simulink model "longitudinal_dynamics"  (R2024b)
settings: Solver=VariableStepAuto  StartTime=0.0  StopTime=60  RelTol=1e-2
values from neighbouring files (symbols this model uses):
  Cd = [0 1]    [mpc3.m]
  Cr = 87342    [mpc3.m]    (also in prueba_mpc.m; prueba_mpc2.m)
  Iz = 1960    [mpc3.m]    (also in prueba_mpc.m; prueba_mpc2.m)
  lf = 1.177    [mpc3.m]    (also in prueba_mpc.m; prueba_mpc2.m)
  lr = 1.358    [mpc3.m]    (also in prueba_mpc.m; prueba_mpc2.m)
  m = 1400    [mpc3.m]    (also in prueba_mpc.m; prueba_mpc2.m)
  R = 1    [prueba_mpc.m]    (also in prueba_mpc2.m)
  vx = 10    [mpc3.m]    (also in prueba_mpc.m; prueba_mpc2.m)
undefined symbols (not defined in the file or in its folder): Af, C_lambda, F_max, FN, g, miu, mode, mu1, mu2, mu3, steering_angle, theta
libraries: mpclib x1, slpidlib x1
settings Model: Creator=inaki  LastModifiedBy=inaki

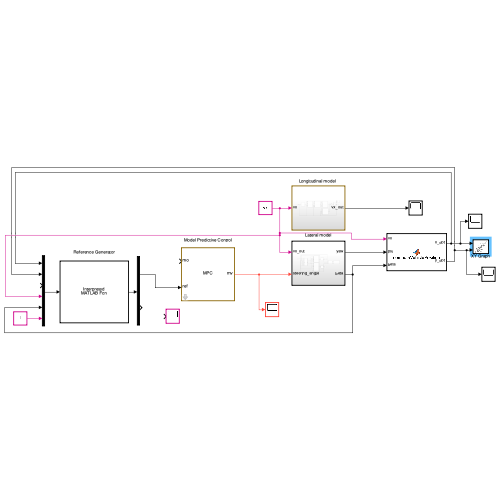
[thumbnail: Simulink's stored preview of the top-level diagram]
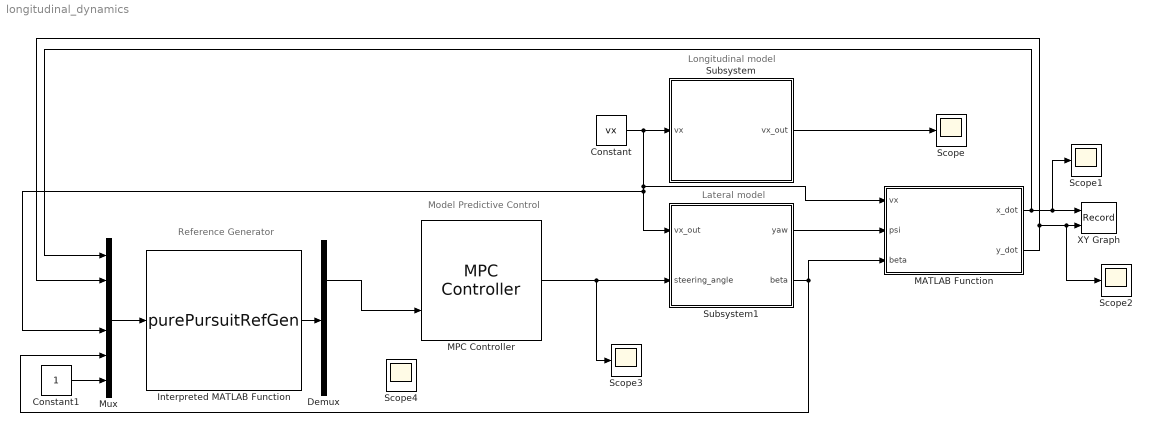
== system longitudinal_dynamics ==
  note: Longitudinal model
  note: Lateral model
  note: Model Predictive Control
  note: Reference Generator
  Constant : Constant  Value=vx
  Constant1 : Constant
  Demux : Demux  Outputs=2
  Interpreted MATLAB Function : MATLABFcn  MATLABFcn=purePursuitRefGen
  MATLAB Function : MATLAB Function  TreatAsAtomicUnit=on
  MPC Controller : mpclib/MPC Controller  SCDEnableBlockLinearizationSpecification=on  mpcobj=mpc1  is_multiple=0  enable_value=0  return_u0=off  updateMPCinCallerWorkspace=on  md_inport=off  mv_inport=off  uref_inport=off  return_cost=off  return_mvseq=off  return_qpstatus=off  return_xseq=off  return_state=off  return_ovseq=off  state_inport=off  umin_inport=off  umax_inport=off  ymin_inport=off  ymax_inport=off  cc_inport=off  ywt_inport=off  uwt_inport=off  duwt_inport=off  rhoeps_inport=off  pm_inport=off  MaximumP=10  HorizonChoice=FixedHorizon  n_ts=0.1  n_p=10  n_mv=1  n_md=0  n_ud=0  n_mo=1  n_uo=0  BlockDataType=double  SampleTimeInherited=off  switch_inport=off
  Mux : Mux  Inputs=6
  Scope{,1..4} (5 alike) : Scope
  Subsystem : Subsystem
  Subsystem1 : Subsystem
  XY Graph : Record  FileSettingsInternal="{\"entries\":[{\"content\":{\"excelSettings\":{\"content\":{},\"type\":\"Streamout.ExcelSettings\"}},\"type\":\"Streamout.FileSettingStorage\",\"uuid\":\"\"}],\"packageUris\":[\"http:\\/\\/schema.mathworks.com\\/mf0\\/streamout_blocks\\/R2020a\"],\"version\":\"1.0\"}"  Layout=[1 1]  SignalsInternal="{\"entries\":[{\"content\":{\"signals\":[{\"content\":{\"blockPath\":[],\"dimensions\":[1],\"domain\":\"\",\"lineColor\":\"#a2142f\",\"plots\":[ 1 ],\"port\":1,\"signalID\":1,\"signalName\":\"MATLAB Function:1\"},\"type\":\"RecordBlkView.Signal\",\"uuid\":\"\"},{\"content\":{\"blockPath\":[],\"dimensions\":[1],\"domain\":\"\",\"lineColor\":\"#139fff\",\"plots\":[ 1 ],\"port\":2,\"signalID\":2,\"signalName\":\"MATLAB Function:2\"},\"type\":\"RecordBlkView.Signal\",\"uuid\":\"\"}]},\"type\":\"RecordBlkView.InputSignals\",\"uuid\":\"\"}],\"packageUris\":[\"http:\\/\\/schema.mathworks.com\\/mf0\\/streamout_blocks\\/R2020a\"],\"version\":\"1.0\"}"  VisualizationBindings="{\"xyplotplugin\":{\"info\":[{\"series\":[{\"bindingParametersList\":[{\"parameter\":\"X-Axis\",\"signalID\":1,\"signalName\":\"MATLAB Function:1\"},{\"parameter\":\"Y-Axis\",\"signalID\":2,\"signalName\":\"MATLAB Function:2\"}],\"seriesID\":0}],\"subplotID\":1}]}}"  CompatibilityTag=XY
  wires:
  Constant/1 -> Subsystem1/1(vx_out), Mux/4, MATLAB Function/1(vx), Subsystem/1(vx)
  Subsystem1/1(yaw) -> MATLAB Function/2(psi)
  Subsystem1/2(beta) -> Mux/5, MATLAB Function/3(beta)
  MATLAB Function/2(y_dot) -> Scope2/1, XY Graph/2, Mux/2
  MATLAB Function/1(x_dot) -> Scope1/1, XY Graph/1, Mux/1
  Interpreted MATLAB Function/1 -> Demux/1
  Demux/1 -> MPC Controller/2
  Mux/1 -> Interpreted MATLAB Function/1
  Constant1/1 -> Mux/6
  MPC Controller/1 -> Scope3/1, Subsystem1/2(steering_angle)
  Subsystem/1(vx_out) -> Scope/1

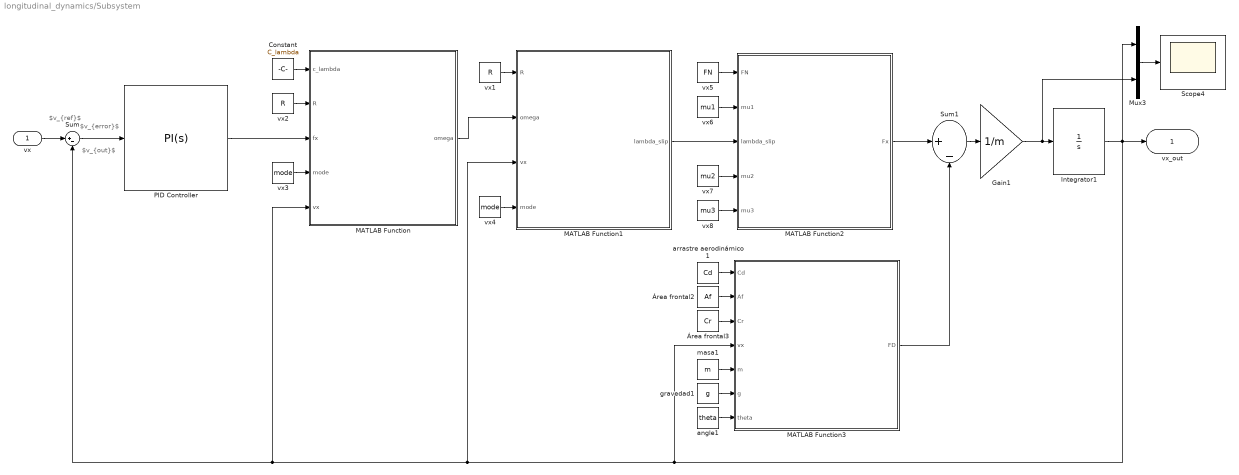
== system longitudinal_dynamics/Subsystem ==
  note: $v_{out}$
  note: $v_{error}$
  note: $v_{ref}$
  vx : Inport
  Constant : Constant  Value=C_lambda
  Gain1 : Gain  Gain=1/m
  Integrator1 : Integrator  ZeroCross=off
  MATLAB Function : MATLAB Function  TreatAsAtomicUnit=on
  MATLAB Function1 : MATLAB Function  TreatAsAtomicUnit=on
  MATLAB Function2 : MATLAB Function  TreatAsAtomicUnit=on
  MATLAB Function3 : MATLAB Function  TreatAsAtomicUnit=on
  Mux3 : Mux  Inputs=2
  PID Controller : slpidlib/PID Controller  Controller=PI  Form=Parallel  TimeDomain=Continuous-time  UseExternalTs=off  SampleTime=-1  IntegratorMethod=Forward Euler  FilterMethod=Forward Euler  ControllerParametersSource=internal  P=3371.8  I=1668.70  UseKiTs=off  D=0  UseExternalDerivativeSource=off  N=100  UseFilter=on  TunerSelectOption=Transfer Function Based (PID Tuner App)  InitialConditionSource=internal  InitialConditionForIntegrator=0  InitialConditionForFilter=0  DifferentiatorICPrevScaledInput=0  ExternalReset=none  TrackingMode=off  Kt=1  LimitOutput=on  SatLimitsSource=internal  UpperSaturationLimit=F_max  LowerSaturationLimit=-F_max  LinearizeAsGain=off  AntiWindupMode=clamping  Kb=1  LimitIntegrator=off  UpperIntegratorSaturationLimit=inf  LowerIntegratorSaturationLimit=-inf  POutMin=[]  POutMax=[]  IOutMin=[]  IOutMax=[]  DOutMin=[]  DOutMax=[]  NOutMin=[]  NOutMax=[]  SumOutMin=[]  SumOutMax=[]  SaturationOutMin=[]  SaturationOutMax=[]  PParamMin=[]  PParamMax=[]  IParamMin=[]  IParamMax=[]  DParamMin=[]  DParamMax=[]  NParamMin=[]  NParamMax=[]  KbParamMin=[]  KbParamMax=[]  KtParamMin=[]  KtParamMax=[]  KbOutMin=[]  KbOutMax=[]  KtOutMin=[]  KtOutMax=[]  IntegratorOutMin=[]  IntegratorOutMax=[]  FilterOutMin=[]  FilterOutMax=[]  SumI1OutMin=[]  SumI1OutMax=[]  SumI2OutMin=[]  SumI2OutMax=[]  SumI3OutMin=[]  SumI3OutMax=[]  SumI4OutMin=[]  SumI4OutMax=[]  SumDOutMin=[]  SumDOutMax=[]  DifferentiatorOutMin=[]  DifferentiatorOutMax=[]  FilterDiffOutCoefMin=[]  FilterDiffOutCoefMax=[]  ReciprocalOutMin=[]  ReciprocalOutMax=[]  SumDenOutMin=[]  SumDenOutMax=[]  SumNumOutMin=[]  SumNumOutMax=[]  DivideOutMin=[]  DivideOutMax=[]  UdiffTsProdOutMin=[]  UdiffTsProdOutMax=[]  NTsProdOutMin=[]  NTsProdOutMax=[]  UintegralTsProdOutMin=[]  UintegralTsProdOutMax=[]  UngainTsProdOutMin=[]  UngainTsProdOutMax=[]  ClampingZeroOutDataTypeStr=Inherit: Inherit via back propagation  ClampingZeroOutMin=[]  ClampingZeroOutMax=[]  FilterDenConstantOutDataTypeStr=Inherit: Inherit via back propagation  FilterDenConstantOutMin=[]  FilterDenConstantOutMax=[]  PCopyOutDataTypeStr=Inherit: Inherit via back propagation  PCopyOutMin=[]  PCopyOutMax=[]  NCopyOutDataTypeStr=Inherit: Inherit via back propagation  NCopyOutMin=[]  NCopyOutMax=[]  IntegratorContinuousStateAttributes=''  IntegratorStateMustResolveToSignalObject=off  IntegratorRTWStateStorageClass=Auto  FilterContinuousStateAttributes=''  FilterStateMustResolveToSignalObject=off  FilterRTWStateStorageClass=Auto  ParallelPVariant=InternalParameters  IdealPVariant=Disabled  IVariant=InternalParameters  DVariant=Disabled  IntegratorVariant=Continuous  SatVariant=Enabled  AWVariant=ContClampingParallel  PCopyVariant=Disabled  TRVariant=Disabled  FdbkBlocksVariant=Forward  IdealPFdbkVariant=Disabled  SatFdbkVariant=Disabled  DerivativeFilterVariant=Disabled  NVariant=Disabled  NCopyVariant=Disabled_SignalSpec  FilterICVariant=Disabled  IntegratorICVariant=InternalICs  ExternalResetVariant=Disabled  TRSumVariant=Passthrough  SumFdbkVariant=Disabled  SumVariant=Sum_PI  TsampFilterVariant=InternalTs  TsampNgainVariant=Passthrough  TsampIntegralVariant=Disabled_SignalSpec  ExternalSaturationOutDataTypeStr=Inherit: Same as second input  DerivativeSourceVariant=Disabled  PreIntVariant=InternalPreInt
  Scope4 : Scope
  Sum : Sum  Inputs=|+-
  Sum1 : Sum  Inputs=|+-
  angle1 : Constant  Value=theta  VectorParams1D=off
  arrastre aerodinámico1 : Constant  Value=Cd  VectorParams1D=off
  gravedad1 : Constant  Value=g  VectorParams1D=off
  masa1 : Constant  Value=m  VectorParams1D=off
  vx1 : Constant  Value=R  VectorParams1D=off  SampleTime=R
  vx2 : Constant  Value=R  VectorParams1D=off  SampleTime=R
  vx3 : Constant  Value=mode  VectorParams1D=off  SampleTime=mode
  vx4 : Constant  Value=mode  VectorParams1D=off  SampleTime=mode
  vx5 : Constant  Value=FN  VectorParams1D=off  SampleTime=R
  vx6 : Constant  Value=mu1  VectorParams1D=off  SampleTime=R
  vx7 : Constant  Value=mu2  VectorParams1D=off  SampleTime=R
  vx8 : Constant  Value=mu3  VectorParams1D=off  SampleTime=R
  Área frontal2 : Constant  Value=Af  VectorParams1D=off
  Área frontal3 : Constant  Value=Cr  VectorParams1D=off
  vx_out : Outport
  wires:
  vx7/1 -> MATLAB Function2/4(mu2)
  vx1/1 -> MATLAB Function1/1(R)
  vx4/1 -> MATLAB Function1/4(mode)
  MATLAB Function3/1(FD) -> Sum1/2
  vx2/1 -> MATLAB Function/2(R)
  gravedad1/1 -> MATLAB Function3/6(g)
  Integrator1/1 -> MATLAB Function/5(vx), Sum/2, MATLAB Function1/3(vx), MATLAB Function3/4(vx), Mux3/1, vx_out/1
  Sum1/1 -> Gain1/1
  Sum/1 -> PID Controller/1
  vx3/1 -> MATLAB Function/4(mode)
  Área frontal2/1 -> MATLAB Function3/2(Af)
  vx6/1 -> MATLAB Function2/2(mu1)
  masa1/1 -> MATLAB Function3/5(m)
  Gain1/1 -> Mux3/2, Integrator1/1
  Constant/1 -> MATLAB Function/1(c_lambda)
  MATLAB Function2/1(Fx) -> Sum1/1
  Mux3/1 -> Scope4/1
  MATLAB Function/1(omega) -> MATLAB Function1/2(omega)
  MATLAB Function1/1(lambda_slip) -> MATLAB Function2/3(lambda_slip)
  vx/1 -> Sum/1
  vx5/1 -> MATLAB Function2/1(FN)
  arrastre aerodinámico1/1 -> MATLAB Function3/1(Cd)
  vx8/1 -> MATLAB Function2/5(mu3)
  angle1/1 -> MATLAB Function3/7(theta)
  PID Controller/1 -> MATLAB Function/3(fx)
  Área frontal3/1 -> MATLAB Function3/3(Cr)

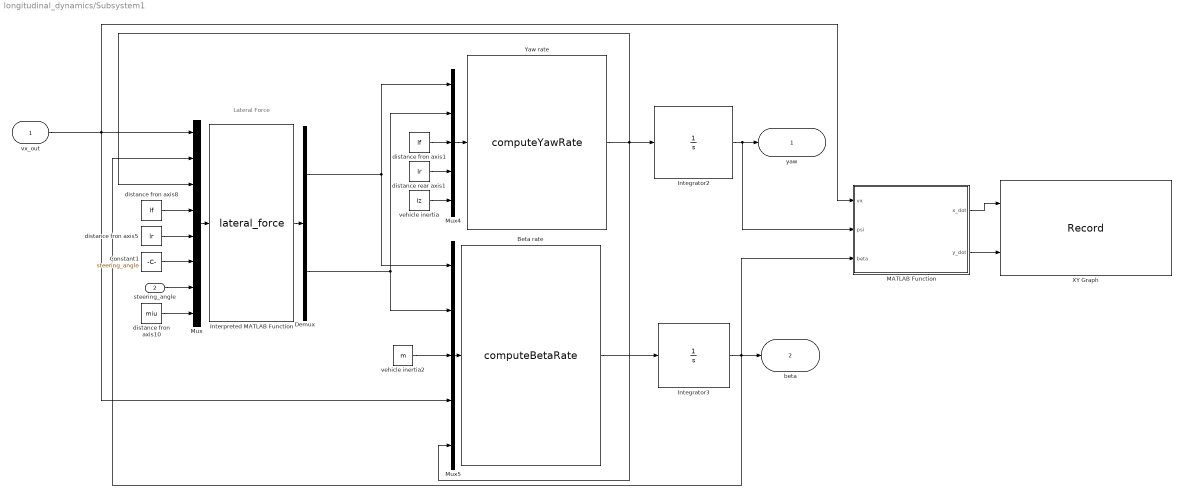
== system longitudinal_dynamics/Subsystem1 ==
  note: Lateral Force
  vx_out : Inport
  steering_angle : Inport  Port=2
  Beta rate : MATLABFcn  MATLABFcn=computeBetaRate
  Constant1 : Constant  Value=steering_angle
  Demux : Demux  Outputs=2
  Integrator2 : Integrator
  Integrator3 : Integrator
  Interpreted MATLAB Function : MATLABFcn  MATLABFcn=lateral_force  OutputDimensions=2
  MATLAB Function : MATLAB Function  TreatAsAtomicUnit=on
  Mux : Mux  Inputs=8
  Mux4 : Mux  Inputs=5
  Mux5 : Mux  Inputs=5
  XY Graph : Record  FileSettingsInternal="{\"entries\":[{\"content\":{\"excelSettings\":{\"content\":{},\"type\":\"Streamout.ExcelSettings\"}},\"type\":\"Streamout.FileSettingStorage\",\"uuid\":\"\"}],\"packageUris\":[\"http:\\/\\/schema.mathworks.com\\/mf0\\/streamout_blocks\\/R2020a\"],\"version\":\"1.0\"}"  Layout=[1 1]  SignalsInternal="{\"entries\":[{\"content\":{\"signals\":[{\"content\":{\"blockPath\":[],\"dimensions\":[1],\"domain\":\"\",\"lineColor\":\"#a2142f\",\"plots\":[ 1 ],\"port\":1,\"signalID\":1,\"signalName\":\"MATLAB Function:1\"},\"type\":\"RecordBlkView.Signal\",\"uuid\":\"\"},{\"content\":{\"blockPath\":[],\"dimensions\":[1],\"domain\":\"\",\"lineColor\":\"#139fff\",\"plots\":[ 1 ],\"port\":2,\"signalID\":2,\"signalName\":\"MATLAB Function:2\"},\"type\":\"RecordBlkView.Signal\",\"uuid\":\"\"}]},\"type\":\"RecordBlkView.InputSignals\",\"uuid\":\"\"}],\"packageUris\":[\"http:\\/\\/schema.mathworks.com\\/mf0\\/streamout_blocks\\/R2020a\"],\"version\":\"1.0\"}"  VisualizationBindings="{\"xyplotplugin\":{\"info\":[{\"series\":[{\"bindingParametersList\":[{\"parameter\":\"X-Axis\",\"signalID\":1,\"signalName\":\"MATLAB Function:1\"},{\"parameter\":\"Y-Axis\",\"signalID\":2,\"signalName\":\"MATLAB Function:2\"}],\"seriesID\":0}],\"subplotID\":1}]}}"  CompatibilityTag=XY
  Yaw rate : MATLABFcn  MATLABFcn=computeYawRate
  distance fron axis1 : Constant  Value=lf
  distance fron axis10 : Constant  Value=miu
  distance fron axis5 : Constant  Value=lr
  distance fron axis8 : Constant  Value=lf
  distance rear axis1 : Constant  Value=lr
  vehicle inertia : Constant  Value=Iz
  vehicle inertia2 : Constant  Value=m
  yaw : Outport
  beta : Outport  Port=2
  wires:
  distance fron axis10/1 -> Mux/8
  distance fron axis8/1 -> Mux/4
  distance fron axis5/1 -> Mux/5
  Constant1/1 -> Mux/6
  steering_angle/1 -> Mux/7
  Demux/1 -> Mux5/1, Mux4/1
  Demux/2 -> Mux5/2, Mux4/2
  vehicle inertia2/1 -> Mux5/3
  Integrator2/1 -> MATLAB Function/2(psi), yaw/1
  Mux4/1 -> Yaw rate/1
  distance rear axis1/1 -> Mux4/4
  distance fron axis1/1 -> Mux4/3
  vehicle inertia/1 -> Mux4/5
  Interpreted MATLAB Function/1 -> Demux/1
  Mux/1 -> Interpreted MATLAB Function/1
  Mux5/1 -> Beta rate/1
  Beta rate/1 -> Integrator3/1
  Yaw rate/1 -> Mux5/5, Integrator2/1, Mux/3
  Integrator3/1 -> Mux/2, beta/1, MATLAB Function/3(beta)
  MATLAB Function/2(y_dot) -> XY Graph/2
  MATLAB Function/1(x_dot) -> XY Graph/1
  vx_out/1 -> Mux5/4, MATLAB Function/1(vx), Mux/1

== matlab function longitudinal_dynamics/Subsystem/MATLAB Function1 ==
  data: R input; lambda_slip output; omega input; vx input; mode input
function lambda_slip = slip_ratio(R,omega,vx,mode)
    epsilon = 1e-6; % Small threshold for near-zero values

    if abs(vx) < epsilon
        vx = sign(vx) * epsilon;
    end
    if abs(omega) < epsilon
        omega = sign(omega) * epsilon;
    end

    if mode == 1  % 'braking'
        if abs(R * omega - vx) < epsilon || abs(vx) < epsilon
            lambda_slip = 0;
        else
            lambda_slip = (R * omega - vx) / vx;
        end
    elseif mode == 2  % 'acceleration'
        if abs(R * omega - vx) < epsilon || abs(R * omega) < epsilon
            lambda_slip = 0;
        else
            lambda_slip = (R * omega - vx) / (R * omega);
        end
    else
        lambda_slip = 1;  
    end
end

== matlab function longitudinal_dynamics/Subsystem/MATLAB Function ==
  data: c_lambda input; R input; fx input; omega output; mode input; vx input
function omega= convertlw(c_lambda, R,fx,  mode,vx)
    % Threshold for near-zero values
    epsilon = 1e-6;
    if abs(fx) < epsilon
        fx = sign(fx) * epsilon;
    end
    if abs(R) < epsilon
        R = sign(R) * epsilon;
    end

    % Compute omega based on mode
    if mode == 1 % braking
        omega = vx * (((fx/c_lambda) +1)/R);
    elseif mode == 2 % acceleration
        omega = (vx*c_lambda) / (R*(c_lambda-fx));
    else
        error('Invalid mode');
    end
end

== matlab function longitudinal_dynamics/Subsystem/MATLAB Function2 ==
  data: FN input; mu1 input; lambda_slip input; Fx output; mu2 input; mu3 input
function Fx = nonlinear_force(FN,mu1,lambda_slip,mu2,mu3)
    mu_lambda = sign(lambda_slip) * (mu1 * (1 - exp(-abs(lambda_slip) * mu2)) - abs(lambda_slip) * mu3);
    Fx = mu_lambda * FN;
end

== matlab function longitudinal_dynamics/Subsystem/MATLAB Function3 ==
  data: Cd input; Af input; Cr input; vx input; FD output; m input; g input; theta input
function FD = drag_force(Cd,Af,Cr,vx,m,g,theta)
    rho = 1.225; 
    drag_term = 0.5 * rho * Cd * Af * vx^2;
    if abs(vx) < 1e-3
        drag_term = 0;  
    end


    rolling_resistance = Cr * m * g * cos(theta);

 
    FD = drag_term + rolling_resistance;


    if ~isfinite(FD)
        FD = 0; 
    end
end

== matlab function longitudinal_dynamics/Subsystem1/MATLAB Function ==
  data: vx input; psi input; x_dot output; beta input; y_dot output
function [x_dot,y_dot] = computeVehiclePosition(vx,psi,beta) 
    vy = vx * tan(beta);
    x_dot = vx * cos(psi) - vy * sin(psi); 
    y_dot = vx * sin(psi) + vy * cos(psi); 

   
end

== matlab function longitudinal_dynamics/MATLAB Function ==
  data: vx input; psi input; x_dot output; beta input; y_dot output
function [x_dot,y_dot] = computeVehiclePosition(vx,psi,beta) 
    vy = vx * tan(beta);
    x_dot = vx * cos(psi) - vy * sin(psi); 
    y_dot = vx * sin(psi) + vy * cos(psi); 

   
end
